simulink model "MotorTest"  (R2017b)
settings: Solver=VariableStepAuto  StartTime=0.0  StopTime=10.0  RelTol=1e-3
undefined symbols (not defined in the file): IC, quadModel
libraries: simulink x2
settings Model: Creator=hoang  LastModifiedBy=hoang

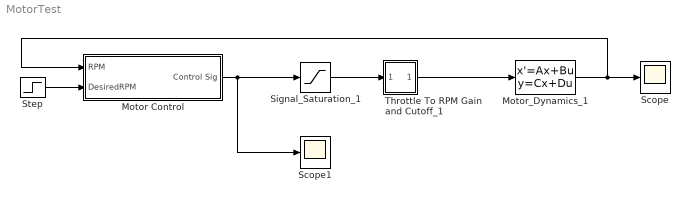
== system MotorTest ==
  Motor Control : Subsystem  mask{k=1.5, Km=quadModel.cr, Ts=1/60, T=quadModel.T, Rdt=100, Rdx=2, b=quadModel.b}
      mask prompts: k "Velocity Gain (k)"; Km "Motor Amplification (Km)"; Ts "Sampling Time (Ts)"; T "Motor Time Constant (T)"; Rdt "Maximum Output Threshold (Rdt)"; Rdx "Maximum Derivative Threshold (Rdx)"; b "Throttle Bias"
      settings: OpenFcn=set_param(gcbh,'LinkStatus','none');
  Motor_Dynamics_1 : StateSpace  A=-1/quadModel.T  C=1/quadModel.T  D=0  InitialCondition=IC.w1*quadModel.T
  Scope : Scope
  Scope1 : Scope
  Signal_Saturation_1 : Saturate  UpperLimit=100  LowerLimit=0
  Step : Step  Before=4000  After=6500  SampleTime=0
  Throttle To RPM Gain and Cutoff_1 : Subsystem
  wires:
  Step/1 -> Motor Control/2(DesiredRPM)
  Signal_Saturation_1/1 -> Throttle To RPM Gain and Cutoff_1/1(In5)
  Throttle To RPM Gain and Cutoff_1/1(Out5) -> Motor_Dynamics_1/1
  Motor Control/1(Control Sig) -> Scope1/1, Signal_Saturation_1/1
  Motor_Dynamics_1/1 -> Motor Control/1(RPM), Scope/1

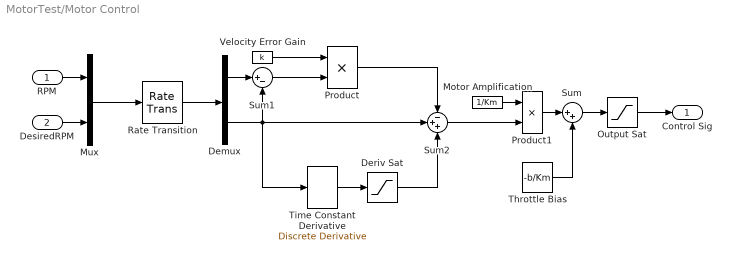
== system MotorTest/Motor Control ==
  RPM : Inport
  DesiredRPM : Inport  Port=2
  Demux : Demux  Outputs=2
  Deriv Sat : Saturate  UpperLimit=Rdx  LowerLimit=-Rdx
  Motor Amplification : Constant  Value=1/Km
  Mux : Mux  Inputs=2
  Output Sat : Saturate  UpperLimit=Rdt  LowerLimit=0
  Product : Product
  Product1 : Product
  Rate Transition : RateTransition  OutPortSampleTime=Ts
  Sum : Sum  Inputs=|++
  Sum1 : Sum  Inputs=|+-
  Sum2 : Sum  Inputs=-++
  Throttle Bias : Constant  Value=-b/Km
  Time Constant Derivative : simulink/Discrete/Discrete Derivative  gainval=T  ICPrevScaledInput=0.0  OutMin=[]  OutMax=[]  OutDataType=fixdt(1, 16)  OutScaling=2^-10  DoSatur=off
  Velocity Error Gain : Constant  Value=k
  Control Sig : Outport
  wires:
  Throttle Bias/1 -> Sum/2
  Sum/1 -> Output Sat/1
  Product1/1 -> Sum/1
  Deriv Sat/1 -> Sum2/3
  Time Constant Derivative/1 -> Deriv Sat/1
  Output Sat/1 -> Control Sig/1
  Motor Amplification/1 -> Product1/1
  Sum2/1 -> Product1/2
  Product/1 -> Sum2/1
  Velocity Error Gain/1 -> Product/1
  Sum1/1 -> Product/2
  Demux/1 -> Sum1/1
  Demux/2 -> Sum1/2, Sum2/2, Time Constant Derivative/1
  Rate Transition/1 -> Demux/1
  Mux/1 -> Rate Transition/1
  DesiredRPM/1 -> Mux/2
  RPM/1 -> Mux/1

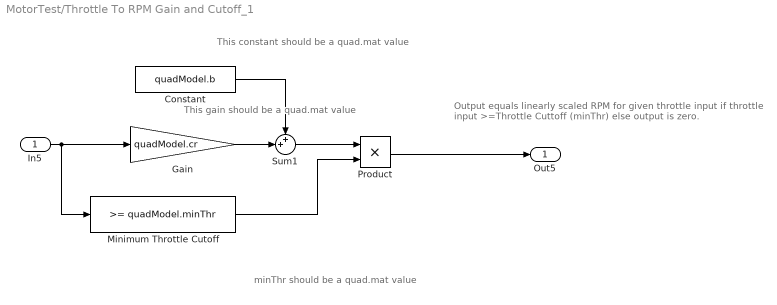
== system MotorTest/Throttle To RPM Gain and Cutoff_1 ==
  note: minThr should be a quad.mat value
  note: This gain should be a quad.mat value
  note: This constant should be a quad.mat value
  note: Output equals linearly scaled RPM
      | for given throttle input if throttle input >=Throttle Cuttoff (minThr)
      | else output is zero.
  In5 : Inport
  Constant : Constant  Value=quadModel.b
  Gain : Gain  Gain=quadModel.cr
  Minimum Throttle Cutoff : simulink/Logic and Bit Operations/Compare To Constant  relop=>=  const=quadModel.minThr  OutDataTypeStr=uint8
  Product : Product
  Sum1 : Sum  Inputs=++|
  Out5 : Outport
  wires:
  Minimum Throttle Cutoff/1 -> Product/2
  Product/1 -> Out5/1
  In5/1 -> Gain/1, Minimum Throttle Cutoff/1
  Gain/1 -> Sum1/2
  Sum1/1 -> Product/1
  Constant/1 -> Sum1/1
